simulink model "zadaca3"  (R2015b)
settings: Solver=FixedStepAuto  StartTime=0.0  StopTime=30  FixedStep=0.001  RelTol=1e-3
libraries: simulink x1
settings Model: Creator=ASIJA  LastModifiedBy=ASIJA

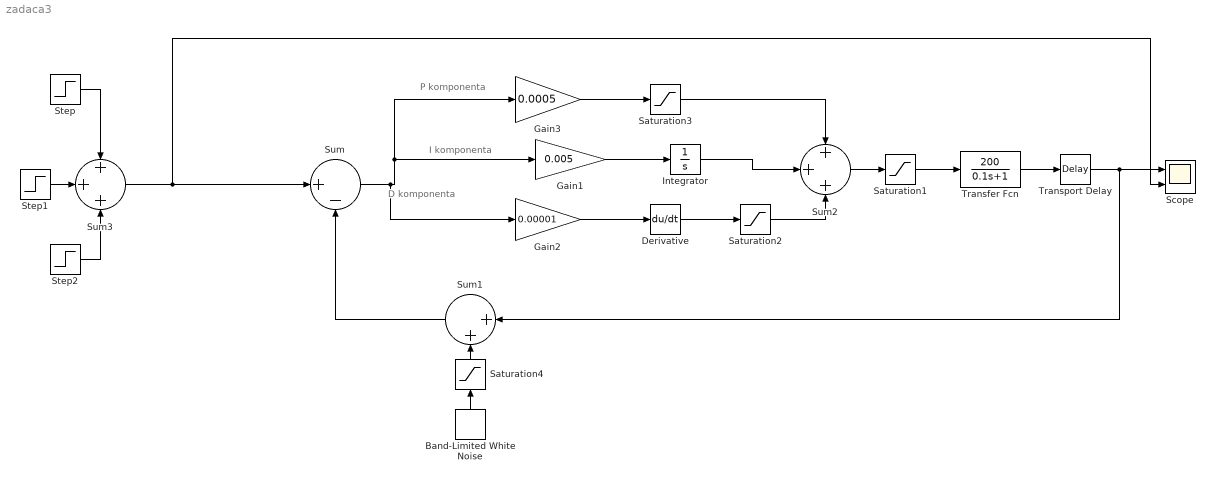
== system zadaca3 ==
  note: P komponenta
  note: D komponenta
  note: I komponenta
  Band-Limited White Noise : simulink/Sources/Band-Limited White Noise  Cov=[0.5]  Ts=0.001  seed=[23341]
  Derivative : Derivative
  Gain1 : Gain  Gain=0.005
  Gain2 : Gain  Gain=0.00001
  Gain3 : Gain  Gain=0.0005
  Integrator : Integrator  LimitOutput=on  UpperSaturationLimit=10  LowerSaturationLimit=0
  Saturation1 : Saturate  UpperLimit=10  LowerLimit=0
  Saturation2 : Saturate  UpperLimit=10  LowerLimit=0
  Saturation3 : Saturate  UpperLimit=10  LowerLimit=0
  Saturation4 : Saturate  LowerLimit=0
  Scope : Scope  NumInputPorts=2
  Step : Step  Time=7  After=80  SampleTime=0
  Step1 : Step  After=45  SampleTime=0
  Step2 : Step  Time=16  Before=57  After=0  SampleTime=0
  Sum : Sum  Inputs=|+-
  Sum1 : Sum  Inputs=|++
  Sum2 : Sum  Inputs=+++
  Sum3 : Sum  Inputs=+++
  Transfer Fcn : TransferFcn  Numerator=[200]  Denominator=[0.1 1]
  Transport Delay : TransportDelay  DelayTime=0.4
  wires:
  Band-Limited White Noise/1 -> Saturation4/1
  Sum1/1 -> Sum/2
  Transfer Fcn/1 -> Transport Delay/1
  Saturation4/1 -> Sum1/2
  Transport Delay/1 -> Sum1/1, Scope/1
  Sum2/1 -> Saturation1/1
  Saturation1/1 -> Transfer Fcn/1
  Gain3/1 -> Saturation3/1
  Saturation3/1 -> Sum2/1
  Gain1/1 -> Integrator/1
  Sum/1 -> Gain2/1, Gain1/1, Gain3/1
  Gain2/1 -> Derivative/1
  Derivative/1 -> Saturation2/1
  Sum3/1 -> Sum/1, Scope/2
  Integrator/1 -> Sum2/2
  Saturation2/1 -> Sum2/3
  Step/1 -> Sum3/1
  Step1/1 -> Sum3/2
  Step2/1 -> Sum3/3
